simulink model "compressor_02_sim"  (R2017b)
settings: Solver=ode23tb  StartTime=0.0  StopTime=tEndSim  MaxStep=1e-1  RelTol=1e-5
values from neighbouring files (symbols this model uses):
  b_motor = 1e-3    (= 0.001)    [compressor_02.m]
  c = conversion_factors()    [compressor_02.m]
  fluid = nh3_v4    [compressor_02.m]
  J_motor = 0.1    [compressor_02.m]
  La_motor = 2.31e-3    (= 0.00231)    [compressor_02.m]
  Ra_motor = 1.5    [compressor_02.m]
  rpm_init = 500    [compressor_02.m]
  slope = (rpm_nominal-rpm_init)/tSweep    (= 4.75)    [compressor_02.m]
undefined symbols (not defined in the file or in its folder): gas, liquid, NH3, P, T
libraries: thermochemical x10, simulink x1
settings Model: Creator=fferrucc  LastModifiedBy=fferrucc

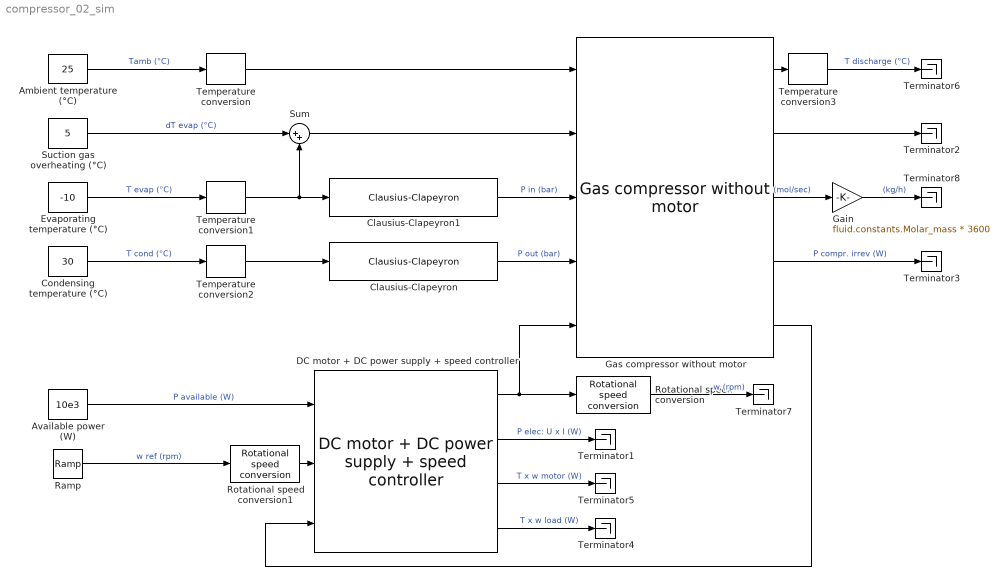
== system compressor_02_sim ==
  Ambient temperature (°C) : Constant  Value=25
  Available power (W) : Constant  Value=10e3
  Clausius-Clapeyron : thermochemical/Thermodynamic fluid properties/Clausius-Clapeyron  sel_1=P(T)  sel_2=NH3(liquid)/NH3(gas)
      settings: SourceProductName=@ Thermochemical
  Clausius-Clapeyron1 : thermochemical/Thermodynamic fluid properties/Clausius-Clapeyron  sel_1=P(T)  sel_2=NH3(liquid)/NH3(gas)
      settings: SourceProductName=@ Thermochemical
  Condensing temperature (°C) : Constant  Value=30
  DC motor + DC power supply + speed controller : thermochemical/Motors/DC motor + DC power supply +  speed controller  L=La_motor  R=Ra_motor  J=J_motor  b=b_motor  Km=Km_motor  w_init_motor=rpm_init*c.rpm_to_rad_sec  PID_P=PID_P_motor  PID_I=PID_I_motor  PID_D=PID_D_motor  V_max=Vmax_motor
      settings: SourceProductName=@ Thermochemical
  Evaporating temperature (°C) : Constant  Value=-10
  Gain : Gain  Gain=fluid.constants.Molar_mass * 3600
  Gas compressor without motor : thermochemical/Compression/Gas compressor without motor  fluid=fluid  eta_IS=eta_IS  CL=CL  eta_mech=eta_mech  dVswept_m3_h=dVswept_m3_h  dVswept_rmp=dVswept_rmp
      settings: SourceProductName=@ Thermochemical
  Ramp : simulink/Sources/Ramp  slope=slope  start=rpm_start_time  X0=rpm_init
  Rotational speed conversion : thermochemical/Conversions/Rotational speed conversion  sel=rad/sec --> rpm
      settings: SourceProductName=@ Thermochemical
  Rotational speed conversion1 : thermochemical/Conversions/Rotational speed conversion  sel=rpm --> rad/sec
      settings: SourceProductName=@ Thermochemical
  Suction gas overheating (°C) : Constant  Value=5
  Sum : Sum  Inputs=|++
  Temperature conversion : thermochemical/Conversions/Temperature conversion  sel=°C --> K
      settings: SourceProductName=@ Thermochemical
  Temperature conversion1 : thermochemical/Conversions/Temperature conversion  sel=°C --> K
      settings: SourceProductName=@ Thermochemical
  Temperature conversion2 : thermochemical/Conversions/Temperature conversion  sel=°C --> K
      settings: SourceProductName=@ Thermochemical
  Temperature conversion3 : thermochemical/Conversions/Temperature conversion  sel=K --> °C
      settings: SourceProductName=@ Thermochemical
  Terminator{1..8} (8 alike) : Terminator
  wires:
  DC motor + DC power supply + speed controller/1 -> Gas compressor without motor/5, Rotational speed conversion/1
  Ambient temperature (°C)/1 -> Temperature conversion/1  "Tamb (°C)"
  Temperature conversion/1 -> Gas compressor without motor/1
  Condensing temperature (°C)/1 -> Temperature conversion2/1  "T cond (°C)"
  Temperature conversion2/1 -> Clausius-Clapeyron/1
  Clausius-Clapeyron/1 -> Gas compressor without motor/4  "P out (bar)"
  Temperature conversion1/1 -> Sum/2, Clausius-Clapeyron1/1
  Evaporating temperature (°C)/1 -> Temperature conversion1/1  "T evap (°C)"
  Clausius-Clapeyron1/1 -> Gas compressor without motor/3  "P in (bar)"
  Sum/1 -> Gas compressor without motor/2
  Suction gas overheating (°C)/1 -> Sum/1  "dT evap (°C)"
  Available power (W)/1 -> DC motor + DC power supply + speed controller/1  "P available (W)"
  Gas compressor without motor/5 -> DC motor + DC power supply + speed controller/3
  Gas compressor without motor/1 -> Temperature conversion3/1
  Temperature conversion3/1 -> Terminator6/1  "T discharge (°C)"
  Gas compressor without motor/3 -> Gain/1  "(mol/sec)"
  Gas compressor without motor/4 -> Terminator3/1  "P compr. irrev (W)"
  DC motor + DC power supply + speed controller/4 -> Terminator4/1  "T x w load (W)"
  DC motor + DC power supply + speed controller/3 -> Terminator5/1  "T x w motor (W)"
  Rotational speed conversion1/1 -> DC motor + DC power supply + speed controller/2
  Rotational speed conversion/1 -> Terminator7/1  "w (rpm)"
  Ramp/1 -> Rotational speed conversion1/1  "w ref (rpm)"
  Gain/1 -> Terminator8/1  "(kg/h)"
  Gas compressor without motor/2 -> Terminator2/1
  DC motor + DC power supply + speed controller/2 -> Terminator1/1  "P elec: U x I (W)"
